simulink model "Pacemaker_OperatingModes"  (R2020a)
settings: Solver=FixedStepAuto  StartTime=0.0  StopTime=10.0  FixedStep=1e-3  RelTol=1e-3  EnableMultiTasking=on
undefined symbols (not defined in the file): A0, A3, D0, D1, D10, D11, D12, D13, D2, D3, D4, D5, D6, D7, D8, D9, PTA0, PTA1, PTA2, PTB11, PTB2, PTB23, PTB9, PTC16, PTC17, PTC2, PTC3, PTC4, PTD0, PTD1, PTD2, PTD3
libraries: frdmk64flib x19
settings Model: ExtModeTrigDuration=5  Creator=furqa  LastModifiedBy=Janahan
settings OptimizationCC: EnhancedBackFolding=on  PassReuseOutputArgsAs=Individual arguments  ZeroExternalMemoryAtStartup=off  ZeroInternalMemoryAtStartup=off  MaxStackSize=64  OptimizeBlockOrder=speed  DifferentSizesBufferReuse=on  OptimizationCustomize=off  EfficientTunableParamExpr=on
settings DebuggingCC: ParameterTunabilityLossMsg=error
settings HardwareCC: ProdBitPerPointer=32  ProdBitPerSizeT=32  ProdBitPerPtrDiffT=32  ProdLargestAtomicInteger=Long  ProdLargestAtomicFloat=Double  ProdWordSize=32  ProdHWDeviceType=ARM Compatible->ARM Cortex
settings SFSimCC: MATLABDynamicMemAlloc=off
settings RTWCC: SystemTargetFile=ert.tlc  HardwareBoard=NXP FRDM-K64F  TemplateMakefile=ert_default_tmf  Toolchain=GNU Tools for ARM Embedded Processors
settings CodeAppCC: ForceParamTrailComments=on  IgnoreCustomStorageClasses=off  OperatorAnnotations=on  SimulinkDataObjDesc=on  SFDataObjDesc=on  InsertBlockDesc=on

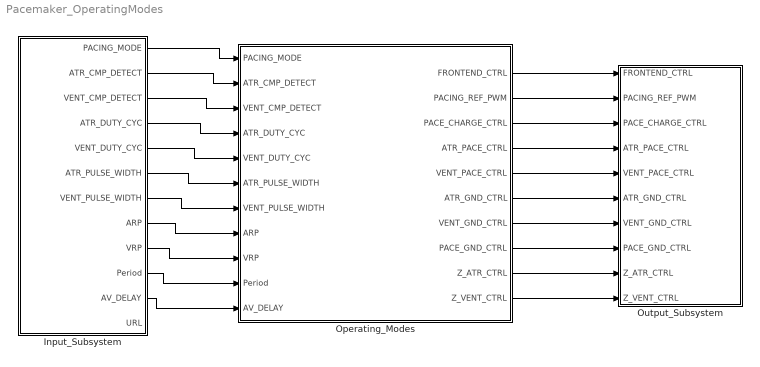
== system Pacemaker_OperatingModes ==
  Input_Subsystem : Subsystem
  Operating_Modes : Stateflow chart  TreatAsAtomicUnit=on
  Output_Subsystem : Subsystem
  wires:
  Input_Subsystem/1(PACING_MODE) -> Operating_Modes/1(PACING_MODE)
  Input_Subsystem/4(ATR_DUTY_CYC) -> Operating_Modes/4(ATR_DUTY_CYC)
  Input_Subsystem/5(VENT_DUTY_CYC) -> Operating_Modes/5(VENT_DUTY_CYC)
  Input_Subsystem/6("ATR_PULSE_WIDTH ") -> Operating_Modes/6(ATR_PULSE_WIDTH)
  Input_Subsystem/7("VENT_PULSE_WIDTH ") -> Operating_Modes/7(VENT_PULSE_WIDTH)
  Operating_Modes/1(FRONTEND_CTRL) -> Output_Subsystem/1(FRONTEND_CTRL)
  Operating_Modes/2(PACING_REF_PWM) -> Output_Subsystem/2(PACING_REF_PWM)
  Operating_Modes/3(PACE_CHARGE_CTRL) -> Output_Subsystem/3(PACE_CHARGE_CTRL)
  Operating_Modes/4(ATR_PACE_CTRL) -> Output_Subsystem/4(ATR_PACE_CTRL)
  Operating_Modes/5(VENT_PACE_CTRL) -> Output_Subsystem/5(VENT_PACE_CTRL)
  Operating_Modes/6(ATR_GND_CTRL) -> Output_Subsystem/6(ATR_GND_CTRL)
  Operating_Modes/7(VENT_GND_CTRL) -> Output_Subsystem/7(VENT_GND_CTRL)
  Operating_Modes/8(PACE_GND_CTRL) -> Output_Subsystem/8(PACE_GND_CTRL)
  Operating_Modes/9(Z_ATR_CTRL) -> Output_Subsystem/9(Z_ATR_CTRL)
  Operating_Modes/10(Z_VENT_CTRL) -> Output_Subsystem/10(Z_VENT_CTRL)
  Input_Subsystem/2(ATR_CMP_DETECT) -> Operating_Modes/2(ATR_CMP_DETECT)
  Input_Subsystem/3(VENT_CMP_DETECT) -> Operating_Modes/3(VENT_CMP_DETECT)
  Input_Subsystem/8(ARP) -> Operating_Modes/8(ARP)
  Input_Subsystem/9(VRP) -> Operating_Modes/9(VRP)
  Input_Subsystem/10("Period ") -> Operating_Modes/10(Period)
  Input_Subsystem/11(AV_DELAY) -> Operating_Modes/11(AV_DELAY)

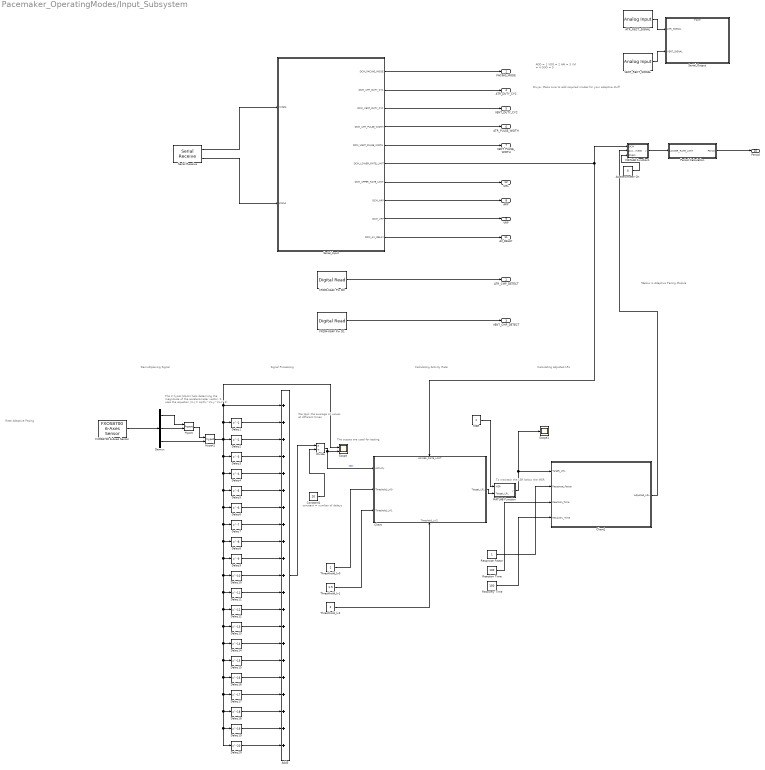
== system Pacemaker_OperatingModes/Input_Subsystem ==
  note: The scopes are used for testing.
  note: The 2 hypot blocks help determing the magnitude of the accelerometer vector. It uses the equation |m| = sqrt(x^2+y^2+z^2)
  note: We took the average of values at different times
  note: To maintain the LSR below the MSR
  note: *Below is Adaptive Pacing Module
  note: Calculating Adjusted LRL
  note: Calculating Activity Rate
  note: Signal Processing
  note: Demultiplexing Signal
  note: Rate Adaptive Pacing
  note: Divya: Make sure to add required modes for your adaptive stuff
  note: AOO = 1
      | VOO = 2
      | AAI = 3
      | VVI = 4
      | DOO = 5
  note: constant = number of delays
  ATR_RECT_SIGNAL : frdmk64flib/Analog Input  Whichpin=PTB11 (A3)  SampleTime=-1
  Accelerometer On : Constant  Value=0
  Add3 : Sum  Inputs=+++++++++++++++++++++
  Chart : Stateflow chart  TreatAsAtomicUnit=on
      settings: PortSchema="{\"entries\":[{\"content\":{\"sides\":[{\"content\":{\"connectorIds\":[\"In4\",\"In3\",\"In1\"]},\"type\":\"ConnectorPlacement.EquallySpacedRectSide\",\"uuid\":\"4cb2c1a3-7832-42b2-9b4d-c3890044bf68\"},{\"content\":{\"connectorIds\":[\"Out1\"],\"side\":\"RIGHT\"},\"type\":\"ConnectorPlacement.EquallySpacedRectSide\",\"uuid\":\"b75defaf-0423-434a-ad80-75ff250baeb0\"},{\"content\":{\"connectorIds\":[\"In5\"],\"side\":\"TOP\"},\"type\":\"ConnectorPlacement.EquallySpacedRectSide\",\"uuid\":\"f36c0704-1900-49b9-9e2d-9f70bdacb700\"},{\"content\":{\"connectorIds\":[\"In2\"],\"side\":\"BOTTOM\"},\"type\":\"ConnectorPlacement.EquallySpacedRectSide\",\"uuid\":\"10402b4c-ca14-4c24-b85b-0c765525471f\"}]},\"type\":\"ConnectorPlacement.EquallySpacedConnector\",\"uuid\":\"93fa6e22-2fd1-4ef1-b7ce-d92ac3f9f3b8\"}],\"packageUris\":[\"http://schema.mathworks.com/mf0/Connector/19700101\"],\"version\":\"1.0\"}"
  Chart1 : Stateflow chart  TreatAsAtomicUnit=on
  Constant1 : Constant  Value=20
  Delay1 : Delay  DelayLength=1
  Delay10 : Delay  DelayLength=10
  Delay11 : Delay  DelayLength=11
  Delay12 : Delay  DelayLength=12
  Delay13 : Delay  DelayLength=13
  Delay14 : Delay  DelayLength=14
  Delay15 : Delay  DelayLength=15
  Delay16 : Delay  DelayLength=16
  Delay17 : Delay  DelayLength=17
  Delay18 : Delay  DelayLength=18
  Delay19 : Delay  DelayLength=19
  Delay2 : Delay
  Delay20 : Delay  DelayLength=20
  Delay3 : Delay  DelayLength=3
  Delay4 : Delay  DelayLength=4
  Delay5 : Delay  DelayLength=5
  Delay6 : Delay  DelayLength=6
  Delay7 : Delay  DelayLength=7
  Delay8 : Delay  DelayLength=8
  Delay9 : Delay  DelayLength=9
  Demux : Demux  Outputs=3
  Divide : Product  Inputs=*/
  FRDM-K64F Pin D0 : frdmk64flib/Digital Read  Whichpin=PTC16 (D0)  SampleTime=-1
  FRDM-K64F Pin D1 : frdmk64flib/Digital Read  Whichpin=PTC17 (D1)  SampleTime=-1
  FXOS8700 6-Axes Sensor : frdmk64flib/FXOS8700 6-Axes Sensor  Activesensor=Accelerometer only  ODR=800Hz  HybridODR=400Hz  Accelfullrange=-4g to +4g  SampleTime=-1
  Hypot : Math  Operator=hypot  SaturateOnIntegerOverflow=on
  Hypot1 : Math  Operator=hypot  SaturateOnIntegerOverflow=on
  MATLAB Function : MATLAB Function  TreatAsAtomicUnit=on
  MATLAB Function1 : MATLAB Function  TreatAsAtomicUnit=on
  MSR : Constant
  Period Calculation : Subsystem
  Reaction Time : Constant  Value=100
  Recovery Time : Constant  Value=150
  Respnose Factor : Constant
  Scope : Scope  NumInputPorts=2
  Scope1 : Scope
  Serial Receive : frdmk64flib/Serial Receive  SCIModule=0  Baudrate=uint32(9600)  Parity=None  StopBits=1  HardwareFlowControl=None  ByteOrder=LittleEndian  DataType=uint8  DataLength=10  BlockingMode=off  OutputStatus=on  SampleTime=0.1
  Serial_Input : Stateflow chart  TreatAsAtomicUnit=on
  Serial_Output : Subsystem
  Threshhold_lv0 : Constant  OutDataTypeStr=double
  Threshhold_lv1 : Constant  Value=1.5
  Threshhold_lv2 : Constant  Value=2
  VENT_RECT_SIGNAL : frdmk64flib/Analog Input  Whichpin=PTB2 (A0)  SampleTime=-1
  PACING_MODE : Outport
  ATR_CMP_DETECT : Outport  Port=2
  VENT_CMP_DETECT : Outport  Port=3
  ATR_DUTY_CYC : Outport  Port=4
  VENT_DUTY_CYC : Outport  Port=5
  "ATR_PULSE_WIDTH " : Outport  Port=6
  "VENT_PULSE_WIDTH " : Outport  Port=7
  ARP : Outport  Port=8
  VRP : Outport  Port=9
  "Period " : Outport  Port=10
  AV_DELAY : Outport  Port=11
  URL : Outport  Port=12
  wires:
  FRDM-K64F Pin D0/1 -> ATR_CMP_DETECT/1
  FRDM-K64F Pin D1/1 -> VENT_CMP_DETECT/1
  Period Calculation/1(Period) -> "Period "/1
  Serial_Input/1(DCM_PACING_MODE) -> PACING_MODE/1
  Serial_Input/2(DCM_ATR_DUTY_CYC) -> ATR_DUTY_CYC/1
  Serial_Input/3(DCM_VENT_DUTY_CYC) -> VENT_DUTY_CYC/1
  Serial_Input/4(DCM_ATR_PULSE_WIDTH) -> "ATR_PULSE_WIDTH "/1
  Serial_Input/5(DCM_VENT_PULSE_WIDTH) -> "VENT_PULSE_WIDTH "/1
  Serial_Input/7(DCM_UPPER_RATE_LIMIT) -> URL/1
  Serial_Input/8(DCM_ARP) -> ARP/1
  Serial_Input/9(DCM_VRP) -> VRP/1
  Serial_Input/10(DCM_AV_DELAY) -> AV_DELAY/1
  Serial Receive/1 -> Serial_Input/1(rxdata)
  Serial Receive/2 -> Serial_Input/2(status)
  ATR_RECT_SIGNAL/1 -> Serial_Output/1(ATR_SIGNAL)
  VENT_RECT_SIGNAL/1 -> Serial_Output/2(VENT_SIGNAL)
  Serial_Input/6(DCM_LOWER_RATE_LIMIT) -> Chart/5(LOWER_RATE_LIMIT), MATLAB Function1/1(DCM)
  Chart1/1(Adjusted_LRL) -> MATLAB Function1/2(Accelerometer)
  Divide/1 -> Chart/4(Activity), Scope/2  "test"
  Recovery Time/1 -> Chart1/4(Recovery_Time)
  Threshhold_lv2/1 -> Chart/2(Threshold_Lvl2)
  Threshhold_lv0/1 -> Chart/3(Threshold_Lvl0)
  Respnose Factor/1 -> Chart1/2(Response_Factor)
  Reaction Time/1 -> Chart1/3(Reaction_Time)
  Delay17/1 -> Add3/18
  Delay11/1 -> Add3/12
  Chart/1(Target_LRL) -> MATLAB Function/2(Target_LRL)
  Demux/2 -> Hypot/2
  Delay10/1 -> Add3/11
  MSR/1 -> MATLAB Function/1(MSR)
  Delay19/1 -> Add3/20
  Delay14/1 -> Add3/15
  Delay12/1 -> Add3/13
  Delay4/1 -> Add3/5
  Hypot/1 -> Hypot1/1
  Delay2/1 -> Add3/3
  Delay1/1 -> Add3/2
  Delay15/1 -> Add3/16
  Delay8/1 -> Add3/9
  Delay7/1 -> Add3/8
  Hypot1/1 -> Delay15/1, Delay19/1, Delay20/1, Delay18/1, Delay17/1, Delay16/1, Delay14/1, Delay13/1, Delay12/1, Delay11/1, Delay10/1, Delay9/1, Delay8/1, Delay7/1, Delay6/1, Delay5/1, Delay4/1, Delay3/1, Delay2/1, Delay1/1, Scope/1, Add3/1
  Constant1/1 -> Divide/2
  Demux/1 -> Hypot/1
  Delay5/1 -> Add3/6
  Delay6/1 -> Add3/7
  Demux/3 -> Hypot1/2
  Delay9/1 -> Add3/10
  Delay13/1 -> Add3/14
  Add3/1 -> Divide/1
  Delay18/1 -> Add3/19
  Delay20/1 -> Add3/21
  FXOS8700 6-Axes Sensor/1 -> Demux/1
  Delay3/1 -> Add3/4
  MATLAB Function/1(y) -> Scope1/1, Chart1/1(Target_LRL)
  Delay16/1 -> Add3/17
  Threshhold_lv1/1 -> Chart/1(Threshold_Lvl1)
  MATLAB Function1/1(y) -> Period Calculation/1(LOWER_RATE_LIMIT)
  Accelerometer On/1 -> MATLAB Function1/3(Check)

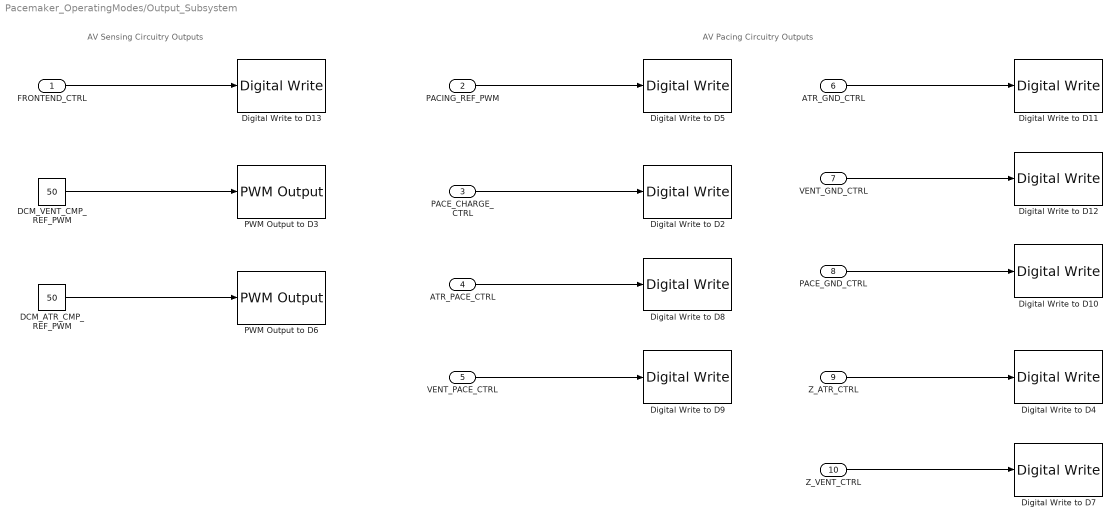
== system Pacemaker_OperatingModes/Output_Subsystem ==
  note: AV Pacing Circuitry Outputs
  note: AV Sensing Circuitry Outputs
  FRONTEND_CTRL : Inport
  PACING_REF_PWM : Inport  Port=2
  PACE_CHARGE_CTRL : Inport  Port=3
  ATR_PACE_CTRL : Inport  Port=4
  VENT_PACE_CTRL : Inport  Port=5
  ATR_GND_CTRL : Inport  Port=6
  VENT_GND_CTRL : Inport  Port=7
  PACE_GND_CTRL : Inport  Port=8
  Z_ATR_CTRL : Inport  Port=9
  Z_VENT_CTRL : Inport  Port=10
  DCM_ATR_CMP_REF_PWM : Constant  Value=50
  DCM_VENT_CMP_REF_PWM : Constant  Value=50
  Digital Write to D10 : frdmk64flib/Digital Write  Whichpin=PTD0 (D10)
  Digital Write to D11 : frdmk64flib/Digital Write  Whichpin=PTD2 (D11)
  Digital Write to D12 : frdmk64flib/Digital Write  Whichpin=PTD3 (D12)
  Digital Write to D13 : frdmk64flib/Digital Write  Whichpin=PTD1 (D13)
  Digital Write to D2 : frdmk64flib/Digital Write  Whichpin=PTB9 (D2)
  Digital Write to D4 : frdmk64flib/Digital Write  Whichpin=PTB23 (D4)
  Digital Write to D5 : frdmk64flib/Digital Write  Whichpin=PTA2 (D5)
  Digital Write to D7 : frdmk64flib/Digital Write  Whichpin=PTC3 (D7)
  Digital Write to D8 : frdmk64flib/Digital Write  Whichpin=PTA0 (D8)
  Digital Write to D9 : frdmk64flib/Digital Write  Whichpin=PTC4 (D9)
  PWM Output to D3 : frdmk64flib/PWM Output  Whichpin=PTA1 (D3)  InitialFrequency=2000  InitialDutyCycle=0
  PWM Output to D6 : frdmk64flib/PWM Output  Whichpin=PTC2 (D6)  InitialFrequency=2000  InitialDutyCycle=0
  wires:
  FRONTEND_CTRL/1 -> Digital Write to D13/1
  DCM_VENT_CMP_REF_PWM/1 -> PWM Output to D3/1
  DCM_ATR_CMP_REF_PWM/1 -> PWM Output to D6/1
  PACING_REF_PWM/1 -> Digital Write to D5/1
  PACE_CHARGE_CTRL/1 -> Digital Write to D2/1
  ATR_PACE_CTRL/1 -> Digital Write to D8/1
  VENT_GND_CTRL/1 -> Digital Write to D12/1
  VENT_PACE_CTRL/1 -> Digital Write to D9/1
  ATR_GND_CTRL/1 -> Digital Write to D11/1
  PACE_GND_CTRL/1 -> Digital Write to D10/1
  Z_ATR_CTRL/1 -> Digital Write to D4/1
  Z_VENT_CTRL/1 -> Digital Write to D7/1

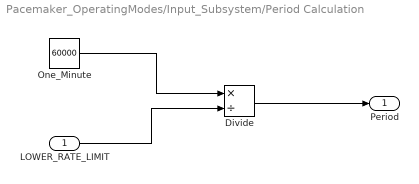
== system Pacemaker_OperatingModes/Input_Subsystem/Period Calculation ==
  LOWER_RATE_LIMIT : Inport
  Divide : Product  Inputs=*/
  One_Minute : Constant  Value=60000
  Period : Outport
  wires:
  One_Minute/1 -> Divide/1
  LOWER_RATE_LIMIT/1 -> Divide/2
  Divide/1 -> Period/1

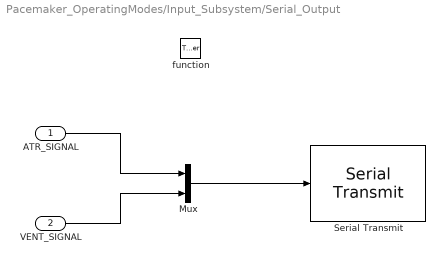
== system Pacemaker_OperatingModes/Input_Subsystem/Serial_Output ==
  ATR_SIGNAL : Inport
  VENT_SIGNAL : Inport  Port=2
  function : TriggerPort  TriggerType=function-call  IsSimulinkFunction=on  FunctionName=send_params  VariantControl=Variant
  Mux : Mux  Inputs=2
  Serial Transmit : frdmk64flib/Serial Transmit  SCIModule=0  Baudrate=uint32(9600)  Parity=None  StopBits=1  HardwareFlowControl=None  ByteOrder=LittleEndian  BlockingMode=on  OutputStatus=off
  wires:
  Mux/1 -> Serial Transmit/1
  VENT_SIGNAL/1 -> Mux/2
  ATR_SIGNAL/1 -> Mux/1

== stateflow chart Pacemaker_OperatingModes/Input_Subsystem/Serial_Input ==
  state SET_PARAMS
    entry:
    DCM_PACING_MODE = typecast(rxdata(4), 'uint8');
    DCM_ATR_DUTY_CYC = typecast(rxdata(5), 'uint8');
    DCM_VENT_DUTY_CYC = typecast(rxdata(6), 'uint8');
    DCM_ATR_PULSE_WIDTH = typecast(rxdata(7), 'uint8');
    DCM_VENT_PULSE_WIDTH = typecast(rxdata(8), 'uint8');
    DCM_LOWER_RATE_LIMIT = typecast(rxdata(9), 'uint8');
    DCM_UPPER_RATE_LIMIT = typecast(rxdata(10), 'uint8');
    DCM_ARP = typecast(rxdata(11:12), 'uint16');
    DCM_VRP = typecast(rxdata(13:14), 'uint16');
    DCM_AV_DELAY = typecast(rxdata(15:16), 'uint16');
  note: This stateflow parses the serial input from the DCM and breaks it down into values to be used by the pacemaker
  state DEFAULT_VALUES
    entry:
    DCM_PACING_MODE = 1;
    DCM_ATR_DUTY_CYC  = 80;
    DCM_VENT_DUTY_CYC  = 80;
    DCM_ATR_PULSE_WIDTH  = 10;
    DCM_VENT_PULSE_WIDTH  = 10;
    DCM_LOWER_RATE_LIMIT  = 60;
    DCM_UPPER_RATE_LIMIT  = 120;
    DCM_ARP  = 250;
    DCM_VRP  = 320;
    DCM_AV_DELAY  = 150;
  state STANDBY
  state SEND_PARAMS
    entry:
    send_param();
  SET_PARAMS -> STANDBY
  (default) -> DEFAULT_VALUES
  (junction 35) -> SET_PARAMS [order 2] : [rxdata(2)==hex2dec('1')]
  (junction 6) -> STANDBY [order 2]
  DEFAULT_VALUES -> STANDBY
  STANDBY -> (junction 6) : [status==0]
  (junction 6) -> (junction 35) [order 1] : [rxdata(1)==hex2dec('33')]
  (junction 35) -> SEND_PARAMS [order 1] : [rxdata(3)==hex2dec('0')]
  data: rxdata input; status input; DCM_PACING_MODE output; DCM_ATR_DUTY_CYC output; DCM_VENT_DUTY_CYC output; DCM_ATR_PULSE_WIDTH output; DCM_VENT_PULSE_WIDTH output; DCM_LOWER_RATE_LIMIT output; DCM_UPPER_RATE_LIMIT output; DCM_ARP output; DCM_VRP output; DCM_AV_DELAY output

== stateflow chart Pacemaker_OperatingModes/Input_Subsystem/Chart ==
  state S_Low
    entry:
    Target_LRL = LOWER_RATE_LIMIT + 5;
  note: The Target LRLs are calculated using restriction in the Activity.
  state S_Medium
    entry:
    Target_LRL = LOWER_RATE_LIMIT +10;
  state S_Rest
    entry:
    Target_LRL = LOWER_RATE_LIMIT;
  state S_Initial
  state S_Medium1
    entry:
    Target_LRL = LOWER_RATE_LIMIT +15;
  S_Initial -> S_Low [order 2] : [Activity >= Threshold_Lvl0 & Activity < Threshold_Lvl1]
  S_Low -> S_Initial
  (default) -> S_Initial
  S_Initial -> S_Medium [order 3] : [Activity >= Threshold_Lvl1 & Activity < Threshold_Lvl2]
  S_Initial -> S_Rest [order 1] : [Activity < Threshold_Lvl0]
  S_Medium -> S_Initial
  S_Rest -> S_Initial
  S_Medium1 -> S_Initial
  S_Initial -> S_Medium1 [order 4] : [Activity >= Threshold_Lvl2]
  data: Threshold_Lvl1 input double; Threshold_Lvl2 input double; Threshold_Lvl0 input double; Target_LRL output double; Activity input double; LOWER_RATE_LIMIT input double

== stateflow chart Pacemaker_OperatingModes/Operating_Modes ==
  state AAI_Pace_OFF
    %These are the pins used to charge the
    % primary capacitors without letting any
    % charge go to the heart
    % This is the charging state
    during:
    ATR_PACE_CTRL= false
    VENT_PACE_CTRL= false
    PACING_REF_PWM= ATR_DUTY_CYC
    PACE_CHARGE_CTRL= true
    PACE_GND_CTRL= true
    Z_ATR_CTRL= false
    Z_VENT_CTRL= false
    ATR_GND_CTRL= true
    VENT_GND_CTRL= false
    FRONTEND_CTRL= true
  state AAI_Pace_ON
    % These pins are used to discharge the primary
    % capacitor into the heart and then zero our
    % voltage using the secondary capacitor.
    % This is the pacing state
    during:
    PACE_CHARGE_CTRL= false
    PACE_GND_CTRL= true
    ATR_PACE_CTRL= true
    ATR_GND_CTRL= false
    Z_ATR_CTRL= false
    Z_VENT_CTRL= false
    VENT_GND_CTRL= false
    VENT_PACE_CTRL= false
    FRONTEND_CTRL= false
  state AAI_Pace_SENSED
    %This state is triggered after sensing a beat
    % This state will be used to incorporate the
    % refractory period as a delay
    during:
    ATR_PACE_CTRL= false
    VENT_PACE_CTRL= false
    PACE_CHARGE_CTRL= true
    PACE_GND_CTRL= true
    Z_ATR_CTRL= false
    Z_VENT_CTRL= false
    ATR_GND_CTRL= true
    VENT_GND_CTRL= false
    FRONTEND_CTRL= false
  state VOO_Pace_OFF
    %These are the pins used to charge the
    % primary capacitors without letting any
    % charge go to the heart
    % This is the charging state
    during:
    ATR_PACE_CTRL = false
    VENT_PACE_CTRL = false
    PACING_REF_PWM =  VENT_DUTY_CYC
    PACE_CHARGE_CTRL = true
    PACE_GND_CTRL = true
    Z_ATR_CTRL = false
    Z_VENT_CTRL = false
    ATR_GND_CTRL = false
    VENT_GND_CTRL = true
    FRONTEND_CTRL = false
  state VOO_Pace_ON
    % These pins are used to discharge the primary
    % capacitor into the heart and then zero our
    % voltage using the secondary capacitor.
    % This is the pacing state
    during:
    PACE_CHARGE_CTRL = false
    PACE_GND_CTRL = true
    ATR_PACE_CTRL = false
    ATR_GND_CTRL = false
    Z_ATR_CTRL = false
    Z_VENT_CTRL = false
    VENT_GND_CTRL = false
    VENT_PACE_CTRL = true
    FRONTEND_CTRL = false
  state VVI_Pace_OFF
    %These are the pins used to charge the
    % primary capacitors without letting any
    % charge go to the heart
    % This is the charging state
    during:
    ATR_PACE_CTRL = false
    VENT_PACE_CTRL = false
    PACING_REF_PWM =  VENT_DUTY_CYC
    PACE_CHARGE_CTRL = true
    PACE_GND_CTRL = true
    Z_ATR_CTRL = false
    Z_VENT_CTRL = false
    ATR_GND_CTRL = false
    VENT_GND_CTRL = true
    FRONTEND_CTRL = true
  state VVI_Pace_SENSED
    %This state is triggered after sensing a beat
    % This state will be used to incorporate the
    % refractory period as a delay
    during:
    ATR_PACE_CTRL = false
    VENT_PACE_CTRL = false
    PACE_CHARGE_CTRL = true
    PACE_GND_CTRL = true
    Z_ATR_CTRL = false
    Z_VENT_CTRL = false
    ATR_GND_CTRL = false
    VENT_GND_CTRL = true
    FRONTEND_CTRL = false
  state VVI_Pace_ON
    % These pins are used to discharge the primary
    % capacitor into the heart and then zero our
    % voltage using the secondary capacitor.
    % This is the pacing state
    during:
    PACE_CHARGE_CTRL = false
    PACE_GND_CTRL = true
    ATR_PACE_CTRL = false
    ATR_GND_CTRL = false
    Z_ATR_CTRL = false
    Z_VENT_CTRL = false
    VENT_GND_CTRL = false
    VENT_PACE_CTRL = true
    FRONTEND_CTRL = false
  state Start
  state AOO_Pace_OFF
    %These are the pins used to charge the
    % primary capacitors without letting any
    % charge go to the heart
    % This is the charging state
    during:
    ATR_PACE_CTRL = false
    VENT_PACE_CTRL = false
    PACING_REF_PWM = ATR_DUTY_CYC
    PACE_CHARGE_CTRL = true
    PACE_GND_CTRL = true
    Z_ATR_CTRL = false
    Z_VENT_CTRL = false
    ATR_GND_CTRL = true
    VENT_GND_CTRL = false
    FRONTEND_CTRL = false
  state AOO_Pace_ON
    % These pins are used to discharge the primary
    % capacitor into the heart and then zero our
    % voltage using the secondary capacitor.
    % This is the pacing state
    during:
    PACE_CHARGE_CTRL = false
    PACE_GND_CTRL = true
    ATR_PACE_CTRL = true
    ATR_GND_CTRL = false
    Z_ATR_CTRL = false
    Z_VENT_CTRL = false
    VENT_GND_CTRL = false
    VENT_PACE_CTRL = false
    FRONTEND_CTRL = false
  state DOO_ATR_Pace_OFF
    %These are the pins used to charge the
    % primary capacitors without letting any
    % charge go to the heart
    % This is the charging state
    during:
    ATR_PACE_CTRL = false
    VENT_PACE_CTRL = false
    PACING_REF_PWM = ATR_DUTY_CYC
    PACE_CHARGE_CTRL = true
    PACE_GND_CTRL = true
    Z_ATR_CTRL = false
    Z_VENT_CTRL = false
    ATR_GND_CTRL = true
    VENT_GND_CTRL = false
    FRONTEND_CTRL = false
  state DOO_ATR_Pace_ON
    % These pins are used to discharge the primary
    % capacitor into the heart and then zero our
    % voltage using the secondary capacitor.
    % This is the pacing state
    during:
    PACE_CHARGE_CTRL = false
    PACE_GND_CTRL = true
    ATR_PACE_CTRL = true
    ATR_GND_CTRL = false
    Z_ATR_CTRL = false
    Z_VENT_CTRL = false
    VENT_GND_CTRL = false
    VENT_PACE_CTRL = false
    FRONTEND_CTRL = false
  state DOO_VENT_Pace_OFF
    %These are the pins used to charge the
    % primary capacitors without letting any
    % charge go to the heart
    % This is the charging state
    during:
    ATR_PACE_CTRL = false
    VENT_PACE_CTRL = false
    PACING_REF_PWM =  VENT_DUTY_CYC
    PACE_CHARGE_CTRL = true
    PACE_GND_CTRL = true
    Z_ATR_CTRL = false
    Z_VENT_CTRL = false
    ATR_GND_CTRL = false
    VENT_GND_CTRL = true
    FRONTEND_CTRL = false
  state DOO_VENT_Pace_ON
    % These pins are used to discharge the primary
    % capacitor into the heart and then zero our
    % voltage using the secondary capacitor.
    % This is the pacing state
    during:
    PACE_CHARGE_CTRL = false
    PACE_GND_CTRL = true
    ATR_PACE_CTRL = false
    ATR_GND_CTRL = false
    Z_ATR_CTRL = false
    Z_VENT_CTRL = false
    VENT_GND_CTRL = false
    VENT_PACE_CTRL = true
    FRONTEND_CTRL = false
  AAI_Pace_ON -> AAI_Pace_SENSED : after(ATR_PULSE_WIDTH,msec)
  (junction 93) -> AAI_Pace_SENSED : after(ATR_PULSE_WIDTH, msec)
  AAI_Pace_OFF -> (junction 93) [order 1] : [ATR_CMP_DETECT==true]
  AAI_Pace_SENSED -> AAI_Pace_OFF : after(ARP,msec)
  AAI_Pace_OFF -> AAI_Pace_ON [order 2] : after(Period - ATR_PULSE_WIDTH - ARP, msec)
  AAI_Pace_OFF -> Start [order 3] : [PACING_MODE~=3]
  Start -> AAI_Pace_OFF [order 4] : [PACING_MODE==3]
  VOO_Pace_ON -> VOO_Pace_OFF : after(Period - VENT_PULSE_WIDTH , msec)
  VOO_Pace_OFF -> Start [order 1] : [PACING_MODE~=2]
  VOO_Pace_OFF -> VOO_Pace_ON [order 2] : after(VENT_PULSE_WIDTH, msec)
  Start -> VOO_Pace_OFF [order 2] : [PACING_MODE == 2]
  (default) -> Start
  Start -> VVI_Pace_OFF [order 5] : [PACING_MODE == 4]
  VVI_Pace_ON -> VVI_Pace_SENSED : after(VENT_PULSE_WIDTH , msec)
  VVI_Pace_OFF -> (junction 91) [order 1] : [VENT_CMP_DETECT==true]
  (junction 91) -> VVI_Pace_SENSED : after(VENT_PULSE_WIDTH, msec)
  VVI_Pace_OFF -> Start [order 2] : [PACING_MODE~=4]
  AOO_Pace_ON -> AOO_Pace_OFF : after(Period - ATR_PULSE_WIDTH, msec)
  VVI_Pace_SENSED -> VVI_Pace_OFF : after(VRP,msec)
  AOO_Pace_OFF -> Start [order 2] : [PACING_MODE ~= 1]
  Start -> AOO_Pace_OFF [order 1] : [PACING_MODE == 1]
  AOO_Pace_OFF -> AOO_Pace_ON [order 1] : after(ATR_PULSE_WIDTH, msec)
  Start -> DOO_ATR_Pace_OFF [order 3] : [PACING_MODE == 5]
  DOO_ATR_Pace_OFF -> Start [order 1] : [PACING_MODE ~= 5]
  VVI_Pace_OFF -> VVI_Pace_ON [order 3] : after(Period - VENT_PULSE_WIDTH - VRP, msec)
  DOO_ATR_Pace_OFF -> DOO_ATR_Pace_ON [order 2] : after(Period - ATR_PULSE_WIDTH - AV_DELAY, msec)
  DOO_ATR_Pace_ON -> DOO_VENT_Pace_OFF : after(ATR_PULSE_WIDTH, msec)
  DOO_VENT_Pace_ON -> DOO_ATR_Pace_OFF : after(Period - VENT_PULSE_WIDTH , msec)
  DOO_VENT_Pace_OFF -> DOO_VENT_Pace_ON : after(AV_DELAY - VENT_PULSE_WIDTH, msec)
  data: FRONTEND_CTRL output; PACING_REF_PWM output; PACE_CHARGE_CTRL output; ATR_PACE_CTRL output; VENT_PACE_CTRL output; ATR_GND_CTRL output; VENT_GND_CTRL output; PACE_GND_CTRL output; Z_ATR_CTRL output; Z_VENT_CTRL output; PACING_MODE input; ATR_CMP_DETECT input; VENT_CMP_DETECT input; ATR_DUTY_CYC input; VENT_DUTY_CYC input; ATR_PULSE_WIDTH input; VENT_PULSE_WIDTH input; ARP input; VRP input; Period input; AV_DELAY input

== stateflow chart Pacemaker_OperatingModes/Input_Subsystem/Chart1 ==
  state Rate_Increase
    entry:
    Adjusted_LRL = Adjusted_LRL + Time*(Target_LRL-Adjusted_LRL)*(1-((0)/((16-Response_Factor)*Reaction_Time)))/Reaction_Time;
    Time = Time + 1;
  state Begin
    entry:
    Adjusted_LRL=Target_LRL;
  state Stay
    entry:
    Time = 0;
  note: ** The time variable makes sure that these 2 logic blocks' running time does not exceed the reaction/recovery time, and the adjusted LRL equations are different respective to if the LRL must be increased or decreased.
  state Rate_Decrease
    during:
    Adjusted_LRL= Adjusted_LRL - Time*(Adjusted_LRL-Target_LRL)*(1-(0)/((16-Response_Factor)*Recovery_Time))/Recovery_Time;
    Time = Time + 1;
  Rate_Increase -> Rate_Increase [order 1] : [Adjusted_LRL<Target_LRL & Time <= Reaction_Time]
  Stay -> Rate_Increase [order 1] : [Adjusted_LRL<Target_LRL]
  (default) -> Begin
  Rate_Increase -> Stay [order 2] : [Adjusted_LRL>=Target_LRL]
  Begin -> Stay
  Rate_Decrease -> Stay [order 2] : [Adjusted_LRL<=Target_LRL]
  Stay -> Rate_Decrease [order 2] : [Adjusted_LRL>Target_LRL]
  Rate_Decrease -> Rate_Decrease [order 1] : [Adjusted_LRL>Target_LRL & Time <= Recovery_Time]
  data: Target_LRL input double; Adjusted_LRL output double; Response_Factor input double; Reaction_Time input double; Recovery_Time input double; Time local double

== matlab function Pacemaker_OperatingModes/Input_Subsystem/MATLAB Function ==
  data: MSR input double; y output double; Target_LRL input double
function y = fcn(MSR, Target_LRL)
    if Target_LRL > MSR
        y=MSR;
    else
        y=Target_LRL;
    end

== matlab function Pacemaker_OperatingModes/Input_Subsystem/MATLAB Function1 ==
  data: y output; DCM input; Accelerometer input; Check input
function y = fcn(DCM, Accelerometer, Check)
    if Check == 0
        y = DCM;
    else
        y = Accelerometer;
    end
